simulink model "SZTAKI_load_and_use_onnx_test"  (R2020b)
settings: Solver=VariableStepAuto  StartTime=0.0  StopTime=1.0  RelTol=1e-3
settings Model: Creator=carmaker-sztaki  LastModifiedBy=carmaker-sztaki

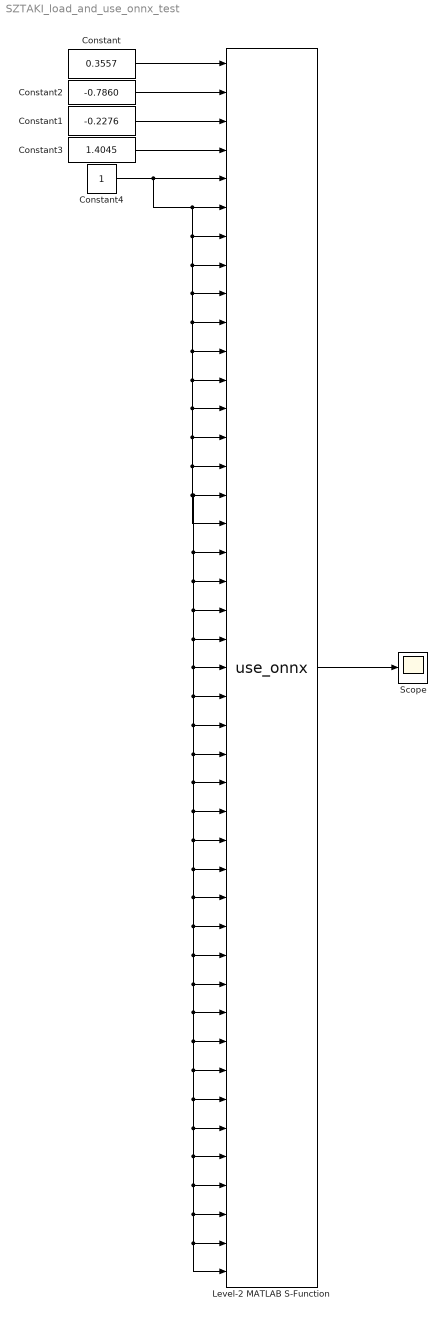
== system SZTAKI_load_and_use_onnx_test ==
  Constant : Constant  Value=0.3557
  Constant1 : Constant  Value=-0.2276
  Constant2 : Constant  Value=-0.7860
  Constant3 : Constant  Value=1.4045
  Constant4 : Constant
  Level-2 MATLAB S-Function : M-S-Function  FunctionName=use_onnx
  Scope : Scope
  wires:
  Constant/1 -> Level-2 MATLAB S-Function/1
  Constant1/1 -> Level-2 MATLAB S-Function/3
  Constant2/1 -> Level-2 MATLAB S-Function/2
  Constant3/1 -> Level-2 MATLAB S-Function/4
  Level-2 MATLAB S-Function/1 -> Scope/1
  Constant4/1 -> Level-2 MATLAB S-Function/17, Level-2 MATLAB S-Function/43, Level-2 MATLAB S-Function/42, Level-2 MATLAB S-Function/41, Level-2 MATLAB S-Function/40, Level-2 MATLAB S-Function/39, Level-2 MATLAB S-Function/38, Level-2 MATLAB S-Function/37, Level-2 MATLAB S-Function/36, Level-2 MATLAB S-Function/35, Level-2 MATLAB S-Function/34, Level-2 MATLAB S-Function/33, Level-2 MATLAB S-Function/32, Level-2 MATLAB S-Function/31, Level-2 MATLAB S-Function/30, Level-2 MATLAB S-Function/29, Level-2 MATLAB S-Function/28, Level-2 MATLAB S-Function/27, Level-2 MATLAB S-Function/26, Level-2 MATLAB S-Function/25, Level-2 MATLAB S-Function/24, Level-2 MATLAB S-Function/23, Level-2 MATLAB S-Function/22, Level-2 MATLAB S-Function/21, Level-2 MATLAB S-Function/20, Level-2 MATLAB S-Function/19, Level-2 MATLAB S-Function/18, Level-2 MATLAB S-Function/16, Level-2 MATLAB S-Function/15, Level-2 MATLAB S-Function/14, Level-2 MATLAB S-Function/13, Level-2 MATLAB S-Function/12, Level-2 MATLAB S-Function/11, Level-2 MATLAB S-Function/10, Level-2 MATLAB S-Function/9, Level-2 MATLAB S-Function/8, Level-2 MATLAB S-Function/7, Level-2 MATLAB S-Function/6, Level-2 MATLAB S-Function/5
